simulink library "orbital_model"  (R2020b)
settings: Solver=VariableStepAuto  StartTime=0.0  StopTime=10.0  RelTol=1e-3
undefined symbols (not defined in the file): mu, r0, v0
libraries: vec_norm x1
settings Model: Creator=whitehole  LastModifiedBy=whitehole

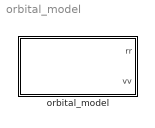
== system orbital_model ==
  orbital_model : Subsystem

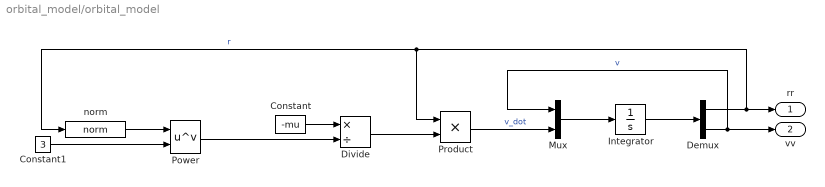
== system orbital_model/orbital_model ==
  Constant : Constant  Value=-mu
  Constant1 : Constant  Value=3
  Demux : Demux  Outputs=2
  Divide : Product  Inputs=*/
  Integrator : Integrator  InitialCondition=[r0 v0]
  Mux : Mux  Inputs=2
  Power : Math  Operator=pow  SaturateOnIntegerOverflow=on
  Product : Product
  norm : vec_norm/norm  SystemSampleTime=-1  VariantActivationTime=update diagram  Latency=0  AutoFrameSizeCalculation=off
  rr : Outport
  vv : Outport  Port=2
  wires:
  Divide/1 -> Product/2
  Mux/1 -> Integrator/1
  Constant/1 -> Divide/1
  Power/1 -> Divide/2
  Product/1 -> Mux/2  "v_dot"
  Integrator/1 -> Demux/1
  Demux/1 -> norm/1, Product/1, rr/1  "r"
  Constant1/1 -> Power/2
  Demux/2 -> Mux/1, vv/1  "v"
  norm/1 -> Power/1
